simulink model "FIR_fda_opt"  (R2015b)
settings: Solver=FixedStepDiscrete  SolverMode=SingleTasking  StartTime=0.0  StopTime=10.0  RelTol=1e-3
libraries: simulink x1
settings Model: Creator=at-mt  LastModifiedBy=amatsumo
settings DataIOCC: SaveFormat=Array  SignalLoggingSaveFormat=ModelDataLogs  SaveOutput=off  SignalLogging=off  SaveTime=off
settings OptimizationCC: BlockReduction=off  ConditionallyExecuteInputs=off  DefaultParameterBehavior=Inlined  ExpressionDepthLimit=2147483647
settings DebuggingCC: AlgebraicLoopMsg=error  UnderspecifiedInitializationDetection=Classic  MergeDetectMultiDrivingBlocksExec=none  SolverPrmCheckMsg=warning  InheritedTsInSrcMsg=none  SingleTaskRateTransMsg=error  FcnCallInpInsideContextMsg=UseLocalSettings  StateNameClashWarn=warning
settings HardwareCC: ProdBitPerPointer=32  ProdLargestAtomicFloat=None  ProdIntDivRoundTo=Undefined  ProdEndianess=Unspecified  ProdWordSize=32  ProdHWDeviceType=ASIC/FPGA->ASIC/FPGA  ProdEqTarget=off
settings GRTTargetCC: GeneratePreprocessorConditionals=Disable all  CombineOutputUpdateFcns=off  GRTInterface=on
settings ConfigComp: CovModelRefEnable=Off  CovSFcnEnable=off

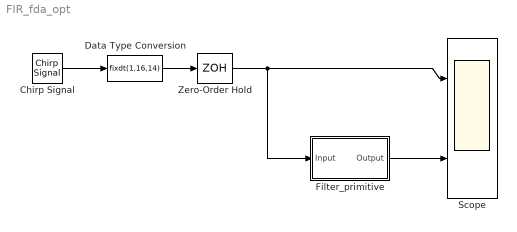
== system FIR_fda_opt ==
  Chirp Signal : simulink/Sources/Chirp Signal  f1=10  T=10  f2=500
  Data Type Conversion : DataTypeConversion  OutDataTypeStr=fixdt(1,16,14)  RndMeth=Nearest
  Filter_primitive : Subsystem  Tag=FilterWizardSubSystem
      settings: ErrorFcn=dspFilterRealizedInBasicElemsAlgLoopErrFcnCallback
  Scope : Scope  NumInputPorts=2
  Zero-Order Hold : ZeroOrderHold  SampleTime=1/1000
  wires:
  Chirp Signal/1 -> Data Type Conversion/1
  Zero-Order Hold/1 -> Scope/1, Filter_primitive/1(Input)
  Data Type Conversion/1 -> Zero-Order Hold/1
  Filter_primitive/1(Output) -> Scope/2

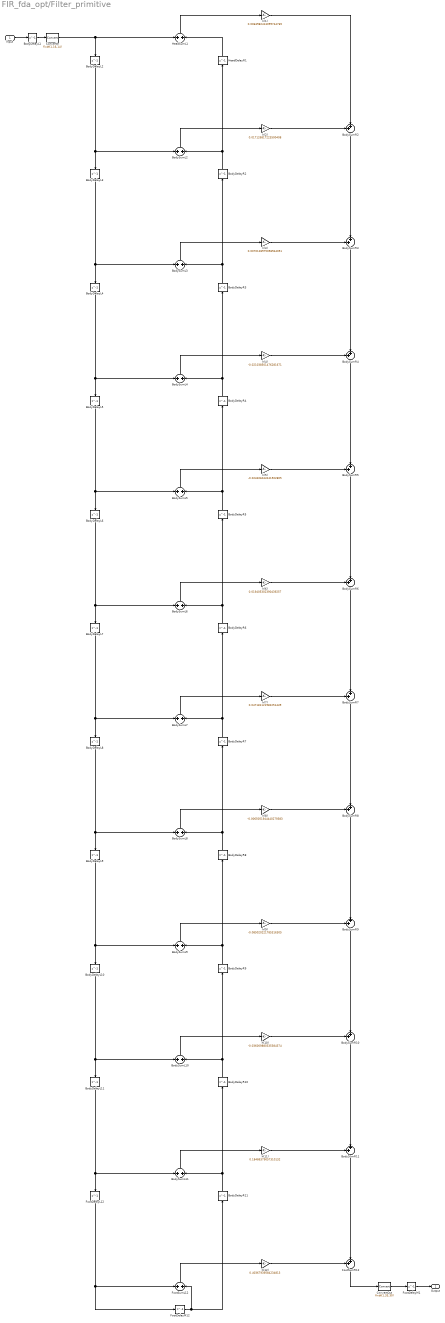
== system FIR_fda_opt/Filter_primitive ==
  Input : Inport
  BodyDelayL{1..11} (11 alike) : Delay  DelayLength=1  InitialCondition=0  InputProcessing=Columns as channels (frame based)
  BodyDelayR{2..11} (10 alike) : Delay  DelayLength=1  InitialCondition=0  InputProcessing=Columns as channels (frame based)
  BodySumL{2..11} (10 alike) : Sum  Inputs=+|+  AccumDataTypeStr=fixdt(1,17,14)  OutDataTypeStr=fixdt(1,17,14)  RndMeth=Convergent
  BodySumR{2..11} (10 alike) : Sum  Inputs=++|  AccumDataTypeStr=fixdt(1,33,30)  OutDataTypeStr=fixdt(1,33,30)  RndMeth=Convergent
  ConvertIn : DataTypeConversion  OutDataTypeStr=fixdt(1,16,14)  RndMeth=Nearest  SaturateOnIntegerOverflow=on
  ConvertOut : DataTypeConversion  OutDataTypeStr=fixdt(1,33,30)  RndMeth=Convergent
  FootDelayL12 : Delay  DelayLength=1  InitialCondition=0  InputProcessing=Columns as channels (frame based)
  FootDelayM1 : Delay  DelayLength=1  InitialCondition=0  InputProcessing=Columns as channels (frame based)
  FootDelayM12 : Delay  DelayLength=1  InitialCondition=0  InputProcessing=Columns as channels (frame based)
  FootSumL12 : Sum  Inputs=+|+  AccumDataTypeStr=fixdt(1,17,14)  OutDataTypeStr=fixdt(1,17,14)  RndMeth=Convergent
  FootSumR12 : Sum  Inputs=++|  AccumDataTypeStr=fixdt(1,33,30)  OutDataTypeStr=fixdt(1,33,30)  RndMeth=Convergent
  HeadDelayR1 : Delay  DelayLength=1  InitialCondition=0  InputProcessing=Columns as channels (frame based)
  HeadSumL1 : Sum  Inputs=+|+  AccumDataTypeStr=fixdt(1,17,14)  OutDataTypeStr=fixdt(1,17,14)  RndMeth=Convergent
  h(1) : Gain  Gain=0.0063982413099744765  ParamDataTypeStr=fixdt(1,16,16)  OutDataTypeStr=fixdt(1,32,30)  RndMeth=Convergent
  h(10) : Gain  Gain=-0.036009880335384374  ParamDataTypeStr=fixdt(1,16,16)  OutDataTypeStr=fixdt(1,32,30)  RndMeth=Convergent
  h(11) : Gain  Gain=0.18486379057310132  ParamDataTypeStr=fixdt(1,16,16)  OutDataTypeStr=fixdt(1,32,30)  RndMeth=Convergent
  h(12) : Gain  Gain=0.40367939584234813  ParamDataTypeStr=fixdt(1,16,16)  OutDataTypeStr=fixdt(1,32,30)  RndMeth=Convergent
  h(2) : Gain  Gain=0.017126817223500408  ParamDataTypeStr=fixdt(1,16,16)  OutDataTypeStr=fixdt(1,32,30)  RndMeth=Convergent
  h(3) : Gain  Gain=0.0070128975058944051  ParamDataTypeStr=fixdt(1,16,16)  OutDataTypeStr=fixdt(1,32,30)  RndMeth=Convergent
  h(4) : Gain  Gain=-0.021038501476281671  ParamDataTypeStr=fixdt(1,16,16)  OutDataTypeStr=fixdt(1,32,30)  RndMeth=Convergent
  h(5) : Gain  Gain=-0.023406043241502805  ParamDataTypeStr=fixdt(1,16,16)  OutDataTypeStr=fixdt(1,32,30)  RndMeth=Convergent
  h(6) : Gain  Gain=0.019405302390439257  ParamDataTypeStr=fixdt(1,16,16)  OutDataTypeStr=fixdt(1,32,30)  RndMeth=Convergent
  h(7) : Gain  Gain=0.047181121982251439  ParamDataTypeStr=fixdt(1,16,16)  OutDataTypeStr=fixdt(1,32,30)  RndMeth=Convergent
  h(8) : Gain  Gain=-0.0065051944440279383  ParamDataTypeStr=fixdt(1,16,16)  OutDataTypeStr=fixdt(1,32,30)  RndMeth=Convergent
  h(9) : Gain  Gain=-0.085020221785316305  ParamDataTypeStr=fixdt(1,16,16)  OutDataTypeStr=fixdt(1,32,30)  RndMeth=Convergent
  Output : Outport
  wires:
  ConvertOut/1 -> FootDelayM1/1
  FootSumR12/1 -> ConvertOut/1
  FootDelayM12/1 -> BodyDelayR11/1, FootSumL12/2
  h(12)/1 -> FootSumR12/1
  FootSumL12/1 -> h(12)/1
  FootDelayL12/1 -> FootDelayM12/1, FootSumL12/1
  BodySumR11/1 -> FootSumR12/2
  BodyDelayR11/1 -> BodyDelayR10/1, BodySumL11/2
  h(11)/1 -> BodySumR11/1
  BodySumL11/1 -> h(11)/1
  BodyDelayL11/1 -> FootDelayL12/1, BodySumL11/1
  BodySumR10/1 -> BodySumR11/2
  BodyDelayR10/1 -> BodyDelayR9/1, BodySumL10/2
  h(10)/1 -> BodySumR10/1
  BodySumL10/1 -> h(10)/1
  BodyDelayL10/1 -> BodyDelayL11/1, BodySumL10/1
  BodySumR9/1 -> BodySumR10/2
  BodyDelayR9/1 -> BodyDelayR8/1, BodySumL9/2
  h(9)/1 -> BodySumR9/1
  BodySumL9/1 -> h(9)/1
  BodyDelayL9/1 -> BodyDelayL10/1, BodySumL9/1
  BodySumR8/1 -> BodySumR9/2
  BodyDelayR8/1 -> BodyDelayR7/1, BodySumL8/2
  h(8)/1 -> BodySumR8/1
  BodySumL8/1 -> h(8)/1
  BodyDelayL8/1 -> BodyDelayL9/1, BodySumL8/1
  BodySumR7/1 -> BodySumR8/2
  BodyDelayR7/1 -> BodyDelayR6/1, BodySumL7/2
  h(7)/1 -> BodySumR7/1
  BodySumL7/1 -> h(7)/1
  BodyDelayL7/1 -> BodyDelayL8/1, BodySumL7/1
  BodySumR6/1 -> BodySumR7/2
  BodyDelayR6/1 -> BodyDelayR5/1, BodySumL6/2
  h(6)/1 -> BodySumR6/1
  BodySumL6/1 -> h(6)/1
  BodyDelayL6/1 -> BodyDelayL7/1, BodySumL6/1
  BodySumR5/1 -> BodySumR6/2
  BodyDelayR5/1 -> BodyDelayR4/1, BodySumL5/2
  h(5)/1 -> BodySumR5/1
  BodySumL5/1 -> h(5)/1
  BodyDelayL5/1 -> BodyDelayL6/1, BodySumL5/1
  BodySumR4/1 -> BodySumR5/2
  BodyDelayR4/1 -> BodyDelayR3/1, BodySumL4/2
  h(4)/1 -> BodySumR4/1
  BodySumL4/1 -> h(4)/1
  BodyDelayL4/1 -> BodyDelayL5/1, BodySumL4/1
  BodySumR3/1 -> BodySumR4/2
  BodyDelayR3/1 -> BodyDelayR2/1, BodySumL3/2
  h(3)/1 -> BodySumR3/1
  BodySumL3/1 -> h(3)/1
  BodyDelayL3/1 -> BodyDelayL4/1, BodySumL3/1
  BodySumR2/1 -> BodySumR3/2
  BodyDelayR2/1 -> HeadDelayR1/1, BodySumL2/2
  h(2)/1 -> BodySumR2/1
  BodySumL2/1 -> h(2)/1
  BodyDelayL2/1 -> BodyDelayL3/1, BodySumL2/1
  ConvertIn/1 -> BodyDelayL2/1, HeadSumL1/1
  HeadDelayR1/1 -> HeadSumL1/2
  h(1)/1 -> BodySumR2/2
  HeadSumL1/1 -> h(1)/1
  Input/1 -> BodyDelayL1/1
  BodyDelayL1/1 -> ConvertIn/1
  FootDelayM1/1 -> Output/1
